simulink model "trans_line_xformer_1"  (Simulink 7.0)
settings: Solver=ode45  StartTime=0.0  StopTime=1e-7  MaxStep=.05e-9;  RelTol=1e-3
libraries: powerlib x9
settings Model: Creator=dbenson  LastModifiedBy=dbenson
settings DebuggingCC: SaveWithParameterizedLinksMsg=none  SignalResolutionControl=TryResolveAllWithWarning  MultiTaskDSMMsg=warning  MultiTaskCondExecSysMsg=none
settings RTWCC: IncludeERTFirstTime=on
settings GRTTargetCC: TargetFcnLib=ansi_tfl_tmw.mat

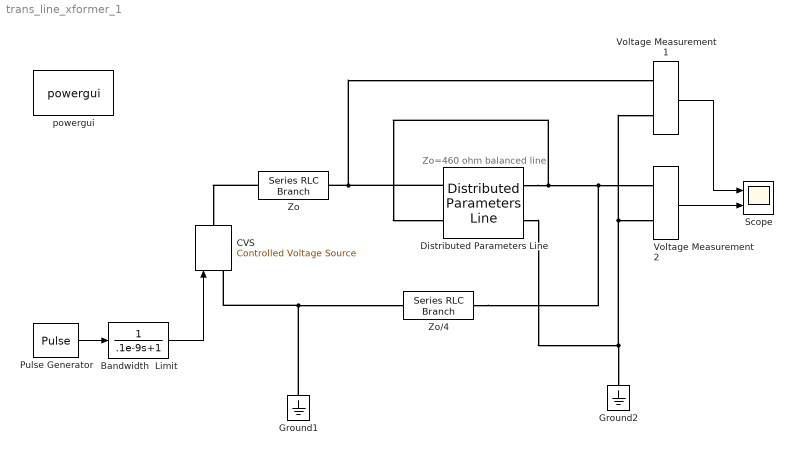
== system trans_line_xformer_1 ==
  note: Zo=460 ohm balanced line
  Bandwidth  Limit : TransferFcn  Denominator=[.1e-9 1]
  CVS : powerlib/Electrical Sources/Controlled Voltage Source  Orientation=up  DialogController=POWERSYS.PowerSysDialog  SystemSampleTime=-1  Initialize=on  Source_Type=DC  Amplitude=0  Phase=0  Frequency=0  Measurements=None
  Distributed Parameters Line : powerlib/Elements/Distributed Parameters Line  DialogController=POWERSYS.PowerSysDialog  SystemSampleTime=-1  Phases=2  Frequency=1000000  Resistance=[33.362 30.175;30.175 33.362]  Inductance=[0.0010569 0.00028823;0.00028823 0.0010569]  Capacitance=[1.141e-008 -3.0743e-009;-3.0743e-009 1.141e-008]  Length=.01  x1=[0 0 0;6.6970441661975e-009 0 0;1.3394088332395e-008 0 0;2.00911324985925e-008 0 0;2.678817666479e-008 0 0;3.34852208309875e-008 0 0]  x2=[0 0 0;6.6970441661975e-009 0 0;1.3394088332395e-008 0 0;2.00911324985925e-008 0 0;2.678817666479e-008 0 0;3.34852208309875e-008 0 0]  x3=[0 0 0;6.6970441661975e-009 0 0;1.3394088332395e-008 0 0;2.00911324985925e-008 0 0;2.678817666479e-008 0 0;3.34852208309875e-008 0 0]  x4=[0 0 0;6.6970441661975e-009 0 0;1.3394088332395e-008 0 0;2.00911324985925e-008 0 0;2.678817666479e-008 0 0;3.34852208309875e-008 0 0]  x5=3.34852208309875e-008  Measurements=None
  Ground1 : powerlib/Elements/Ground  Orientation=down  DialogController=POWERSYS.PowerSysDialog  PhysicalDomain=powersysdomain  SubClassName=unknown  LeftPortType=p1  RightPortType=p1  LConnTagsString=a
  Ground2 : powerlib/Elements/Ground  Orientation=down  DialogController=POWERSYS.PowerSysDialog  PhysicalDomain=powersysdomain  SubClassName=unknown  LeftPortType=p1  RightPortType=p1  LConnTagsString=a
  Pulse Generator : DiscretePulseGenerator  PulseType=Time based  Period=0.5e-7  PulseWidth=50
  Scope : Scope  NumInputPorts=2
      settings: YMin=-5~-5  YMax=5~5
  Voltage Measurement1 : powerlib/Measurements/Voltage Measurement  DialogController=POWERSYS.PowerSysDialog  SystemSampleTime=-1  PhasorSimulation=off  OutputType=Complex  PSBequivalent=0
  Voltage Measurement2 : powerlib/Measurements/Voltage Measurement  DialogController=POWERSYS.PowerSysDialog  SystemSampleTime=-1  PhasorSimulation=off  OutputType=Complex  PSBequivalent=0
  Zo : powerlib/Elements/Series RLC Branch  DialogController=POWERSYS.PowerSysDialog  PhysicalDomain=powersysdomain  SubClassName=unknown  LeftPortType=p1  RightPortType=p1  LConnTagsString=__new0  RConnTagsString=__new0  BranchType=R  Resistance=460.7  Inductance=1e-3  SetiL0=off  InitialCurrent=0  Capacitance=1e-6  Setx0=off  InitialVoltage=0  Measurements=None
  Zo/4 : powerlib/Elements/Series RLC Branch  DialogController=POWERSYS.PowerSysDialog  PhysicalDomain=powersysdomain  SubClassName=unknown  LeftPortType=p1  RightPortType=p1  LConnTagsString=__new0  RConnTagsString=__new0  BranchType=R  Resistance=460.7/4  Inductance=1e-3  SetiL0=off  InitialCurrent=0  Capacitance=1e-6  Setx0=off  InitialVoltage=0  Measurements=None
  powergui : powerlib/powergui  SystemSampleTime=-1  SimulationMode=Continuous  SampleTime=50e-6  echomessages=off  RestoreLinks=warning  x0status=blocks  Frange=[0:2:500]  Ylog=off  Xlog=on  ShowGrid=off  save=off  variable=ZData  ZoomFFT=on  StartTime=0.0  cycles=1  DisplayStyle=1  fundamental=60  FreqAxis=off  MaxFrequency=1000  frequencyindice=0  frequencyindicesteady=1  RmsSteady=1  display=off  Ts=0  frequency=60  methode=off  HookPort=off  Interpol=off  SPID=off  FunctionMessages=off
  wires:
  Pulse Generator/1 -> Bandwidth  Limit/1
  Bandwidth  Limit/1 -> CVS/1
  Voltage Measurement2/1 -> Scope/2
  Voltage Measurement1/1 -> Scope/1
  connections:
  Distributed Parameters Line/LConn1 -- Zo/RConn1 -- Voltage Measurement1/LConn1
  Zo/LConn1 -- CVS/RConn1
  Distributed Parameters Line/RConn1 -- Distributed Parameters Line/LConn2 -- Voltage Measurement2/LConn1 -- Zo/4/RConn1
  CVS/LConn1 -- Ground1/LConn1 -- Zo/4/LConn1
  Distributed Parameters Line/RConn2 -- Ground2/LConn1 -- Voltage Measurement2/LConn2 -- Voltage Measurement1/LConn2
